simulink model "gm_Qiu_YQ"  (R2020a)
settings: Solver=FixedStepDiscrete  StartTime=0.0  StopTime=1.5  RelTol=1e-3
undefined symbols (not defined in the file or in its folder): N
libraries: dspsrcs4 x1
settings Model: SimulationMode=accelerator  Creator=huawei  LastModifiedBy=huawei
settings DataIOCC: SaveOutput=off  SaveTime=off
settings OptimizationCC: BlockReduction=off  ConditionallyExecuteInputs=off  DefaultParameterBehavior=Inlined
settings DebuggingCC: SignalRangeChecking=error  AlgebraicLoopMsg=error  InheritedTsInSrcMsg=none  SingleTaskRateTransMsg=error  ParameterDowncastMsg=none  ParameterOverflowMsg=none  ParameterPrecisionLossMsg=none  ArithmeticOperatorsInVariantConditions=warning
settings HardwareCC: ProdBitPerPointer=32  ProdBitPerSizeT=32  ProdBitPerPtrDiffT=32  ProdLargestAtomicFloat=None  ProdIntDivRoundTo=Undefined  ProdEndianess=Unspecified  ProdWordSize=32  ProdHWDeviceType=ASIC/FPGA->ASIC/FPGA  TargetBitPerPointer=64  TargetBitPerSizeT=64  TargetBitPerPtrDiffT=64  TargetLongLongMode=on  TargetIntDivRoundTo=Zero  TargetEndianess=LittleEndian  TargetWordSize=64  TargetHWDeviceType=Custom Processor->MATLAB Host Computer  ProdEqTarget=off
settings SFSimCC: CustomCodeUndefinedFunction=UseInterfaceOnly

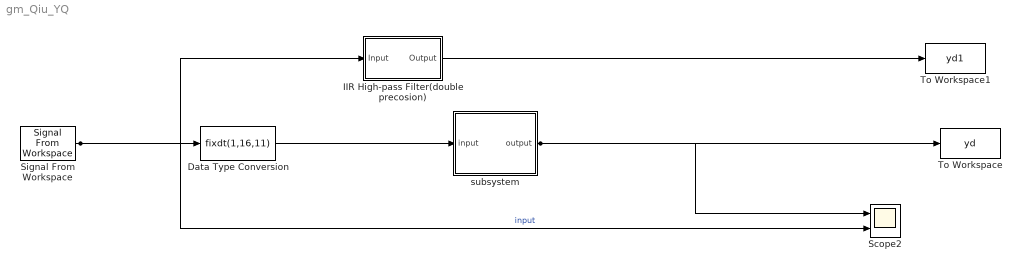
== system gm_Qiu_YQ ==
  Data Type Conversion : DataTypeConversion  OutDataTypeStr=fixdt(1,16,11)  RndMeth=Convergent
  IIR High-pass Filter(double precosion) : Subsystem  Tag=FilterWizardSubSystem
      settings: ErrorFcn=dspFilterRealizedInBasicElemsAlgLoopErrFcnCallback
  Scope2 : Scope  NumInputPorts=2
  Signal From Workspace : dspsrcs4/Signal From Workspace  X=x  Ts=1/N  nsamps=1  OutputAfterFinalValue=Setting to zero  ignoreOrWarnInputAndFrameLengths=off  OutputFrames=off
  To Workspace : ToWorkspace  VariableName=yd  SaveFormat=Timeseries  SampleTime=-1
  To Workspace1 : ToWorkspace  VariableName=yd1  SaveFormat=Timeseries  SampleTime=-1
  subsystem : Subsystem
  wires:
  Data Type Conversion/1 -> subsystem/1(input)
  subsystem/1(output) -> To Workspace/1, Scope2/1
  IIR High-pass Filter(double precosion)/1(Output) -> To Workspace1/1
  Signal From Workspace/1 -> Data Type Conversion/1, IIR High-pass Filter(double precosion)/1(Input), Scope2/2  "input"

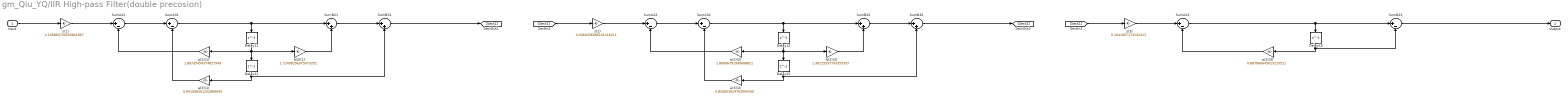
== system gm_Qiu_YQ/IIR High-pass Filter(double precosion) ==
  Input : Inport
  Delay{11..13,21..22} (5 alike) : Delay  DelayLength=1  InitialCondition=0
  SumA{21..23,31..32} (5 alike) : Sum  Inputs=|+-  RndMeth=Nearest  SaturateOnIntegerOverflow=on  OutDataTypeStr=Inherit: Same as first input
  SumB{21..22,31..32} (4 alike) : Sum  Inputs=|++  RndMeth=Nearest  SaturateOnIntegerOverflow=on  OutDataTypeStr=Inherit: Same as first input
  SumB23 : Sum  Inputs=|+-  RndMeth=Nearest  SaturateOnIntegerOverflow=on  OutDataTypeStr=Inherit: Same as first input
  a(2)(1) : Gain  Gain=1.88735454374827949  ParamDataTypeStr=double  RndMeth=Nearest  SaturateOnIntegerOverflow=on  OutDataTypeStr=Inherit: Same as input
  a(2)(2) : Gain  Gain=1.80696791990688821  ParamDataTypeStr=double  RndMeth=Nearest  SaturateOnIntegerOverflow=on  OutDataTypeStr=Inherit: Same as input
  a(2)(3) : Gain  Gain=0.887060645613220511  ParamDataTypeStr=double  RndMeth=Nearest  SaturateOnIntegerOverflow=on  OutDataTypeStr=Inherit: Same as input
  a(3)(1) : Gain  Gain=0.941058301252869045  ParamDataTypeStr=double  RndMeth=Nearest  SaturateOnIntegerOverflow=on  OutDataTypeStr=Inherit: Same as input
  a(3)(2) : Gain  Gain=0.835803624763594266  ParamDataTypeStr=double  RndMeth=Nearest  SaturateOnIntegerOverflow=on  OutDataTypeStr=Inherit: Same as input
  b(2)(1) : Gain  Gain=1.72499296375073352  ParamDataTypeStr=double  RndMeth=Nearest  SaturateOnIntegerOverflow=on  OutDataTypeStr=Inherit: Same as input
  b(2)(2) : Gain  Gain=1.38125597793355337  ParamDataTypeStr=double  RndMeth=Nearest  SaturateOnIntegerOverflow=on  OutDataTypeStr=Inherit: Same as input
  s(1) : Gain  Gain=0.105863730533801867  ParamDataTypeStr=double  RndMeth=Nearest  SaturateOnIntegerOverflow=on  OutDataTypeStr=Inherit: Same as input
  s(2) : Gain  Gain=0.0466036096161416211  ParamDataTypeStr=double  RndMeth=Nearest  SaturateOnIntegerOverflow=on  OutDataTypeStr=Inherit: Same as input
  s(3) : Gain  Gain=0.1041667174132411  ParamDataTypeStr=double  RndMeth=Nearest  SaturateOnIntegerOverflow=on  OutDataTypeStr=Inherit: Same as input
  Output : Outport
  wires:
  Delay13/1 -> SumB23/2, a(2)(3)/1
  a(2)(3)/1 -> SumA23/2
  SumB23/1 -> Output/1
  SumA23/1 -> Delay13/1, SumB23/1
  s(3)/1 -> SumA23/1
  [Sect2] -> s(3)/1
  Delay22/1 -> SumB32/2, a(3)(2)/1
  a(3)(2)/1 -> SumA32/2
  b(2)(2)/1 -> SumB22/2
  Delay12/1 -> Delay22/1, b(2)(2)/1, a(2)(2)/1
  a(2)(2)/1 -> SumA22/2
  SumB32/1 -> [Sect2]
  SumB22/1 -> SumB32/1
  SumA32/1 -> Delay12/1, SumB22/1
  SumA22/1 -> SumA32/1
  s(2)/1 -> SumA22/1
  [Sect1] -> s(2)/1
  Delay21/1 -> SumB31/2, a(3)(1)/1
  a(3)(1)/1 -> SumA31/2
  b(2)(1)/1 -> SumB21/2
  Delay11/1 -> Delay21/1, b(2)(1)/1, a(2)(1)/1
  a(2)(1)/1 -> SumA21/2
  SumB31/1 -> [Sect1]
  SumB21/1 -> SumB31/1
  SumA31/1 -> Delay11/1, SumB21/1
  SumA21/1 -> SumA31/1
  s(1)/1 -> SumA21/1
  Input/1 -> s(1)/1

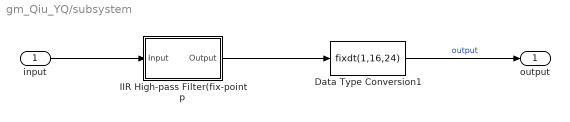
== system gm_Qiu_YQ/subsystem ==
  input : Inport
  Data Type Conversion1 : DataTypeConversion  OutDataTypeStr=fixdt(1,16,24)
  IIR High-pass Filter(fix-point p : Subsystem  Tag=FilterWizardSubSystem
      settings: ErrorFcn=dspFilterRealizedInBasicElemsAlgLoopErrFcnCallback
  output : Outport
  wires:
  Data Type Conversion1/1 -> output/1  "output"
  input/1 -> IIR High-pass Filter(fix-point p/1(Input)
  IIR High-pass Filter(fix-point p/1(Output) -> Data Type Conversion1/1

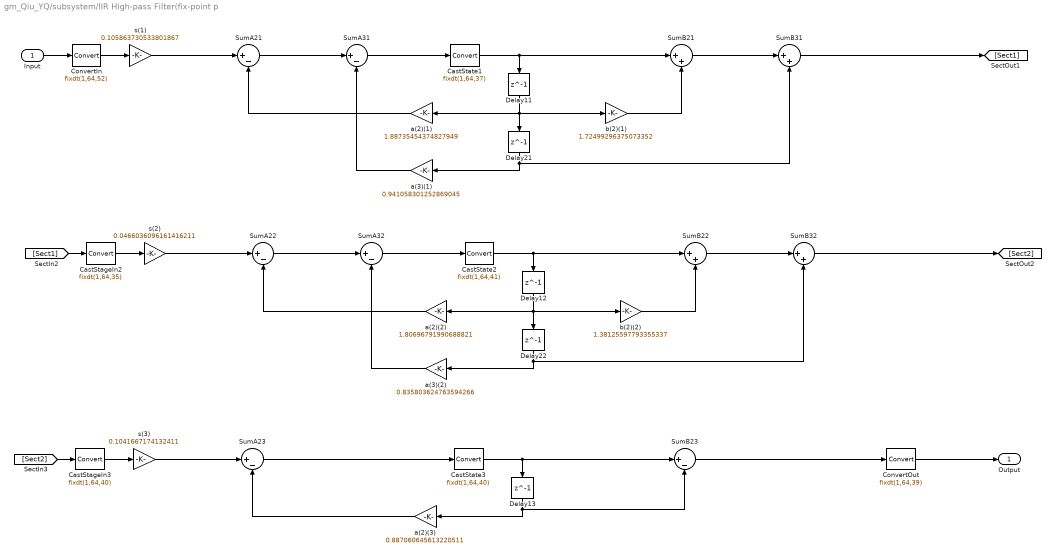
== system gm_Qiu_YQ/subsystem/IIR High-pass Filter(fix-point p ==
  Input : Inport  OutDataTypeStr=fixdt(1,16,11)  LockScale=on
  CastStageIn2 : DataTypeConversion  OutDataTypeStr=fixdt(1,64,35)  RndMeth=Convergent
  CastStageIn3 : DataTypeConversion  OutDataTypeStr=fixdt(1,64,40)  RndMeth=Convergent
  CastState1 : DataTypeConversion  OutDataTypeStr=fixdt(1,64,37)  RndMeth=Convergent
  CastState2 : DataTypeConversion  OutDataTypeStr=fixdt(1,64,41)  RndMeth=Convergent
  CastState3 : DataTypeConversion  OutDataTypeStr=fixdt(1,64,40)  RndMeth=Convergent
  ConvertIn : DataTypeConversion  OutDataTypeStr=fixdt(1,64,52)  RndMeth=Nearest  SaturateOnIntegerOverflow=on
  ConvertOut : DataTypeConversion  OutDataTypeStr=fixdt(1,64,39)  RndMeth=Convergent
  Delay{11..13,21..22} (5 alike) : Delay  DelayLength=1  InitialCondition=0
  SumA21 : Sum  Inputs=|+-  AccumDataTypeStr=fixdt(1,64,53)  OutDataTypeStr=fixdt(1,64,33)  RndMeth=Convergent
  SumA22 : Sum  Inputs=|+-  AccumDataTypeStr=fixdt(1,64,39)  OutDataTypeStr=fixdt(1,64,37)  RndMeth=Convergent
  SumA23 : Sum  Inputs=|+-  AccumDataTypeStr=fixdt(1,64,39)  OutDataTypeStr=fixdt(1,64,39)  RndMeth=Convergent
  SumA31 : Sum  Inputs=|+-  AccumDataTypeStr=fixdt(1,64,33)  OutDataTypeStr=fixdt(1,64,34)  RndMeth=Convergent
  SumA32 : Sum  Inputs=|+-  AccumDataTypeStr=fixdt(1,64,37)  OutDataTypeStr=fixdt(1,64,38)  RndMeth=Convergent
  SumB21 : Sum  Inputs=|++  AccumDataTypeStr=fixdt(1,64,33)  OutDataTypeStr=fixdt(1,64,33)  RndMeth=Convergent
  SumB22 : Sum  Inputs=|++  AccumDataTypeStr=fixdt(1,64,38)  OutDataTypeStr=fixdt(1,64,38)  RndMeth=Convergent
  SumB23 : Sum  Inputs=|+-  AccumDataTypeStr=fixdt(1,64,39)  OutDataTypeStr=fixdt(1,64,39)  RndMeth=Convergent
  SumB31 : Sum  Inputs=|++  AccumDataTypeStr=fixdt(1,64,35)  OutDataTypeStr=fixdt(1,64,34)  RndMeth=Convergent
  SumB32 : Sum  Inputs=|++  AccumDataTypeStr=fixdt(1,64,38)  OutDataTypeStr=fixdt(1,64,37)  RndMeth=Convergent
  a(2)(1) : Gain  Gain=1.88735454374827949  ParamDataTypeStr=fixdt(0,16,15)  OutDataTypeStr=fixdt(1,64,32)  RndMeth=Convergent
  a(2)(2) : Gain  Gain=1.80696791990688821  ParamDataTypeStr=fixdt(0,16,15)  OutDataTypeStr=fixdt(1,32,35)  RndMeth=Convergent
  a(2)(3) : Gain  Gain=0.887060645613220511  ParamDataTypeStr=fixdt(0,16,16)  OutDataTypeStr=fixdt(1,32,38)  RndMeth=Convergent
  a(3)(1) : Gain  Gain=0.941058301252869045  ParamDataTypeStr=fixdt(0,16,16)  OutDataTypeStr=fixdt(1,64,34)  RndMeth=Convergent
  a(3)(2) : Gain  Gain=0.835803624763594266  ParamDataTypeStr=fixdt(0,16,16)  OutDataTypeStr=fixdt(1,32,36)  RndMeth=Convergent
  b(2)(1) : Gain  Gain=1.72499296375073352  ParamDataTypeStr=fixdt(0,16,15)  OutDataTypeStr=fixdt(1,64,34)  RndMeth=Convergent
  b(2)(2) : Gain  Gain=1.38125597793355337  ParamDataTypeStr=fixdt(0,16,15)  OutDataTypeStr=fixdt(1,32,35)  RndMeth=Convergent
  s(1) : Gain  Gain=0.105863730533801867  ParamDataTypeStr=fixdt(0,16,19)  OutDataTypeStr=fixdt(1,64,54)  RndMeth=Convergent
  s(2) : Gain  Gain=0.0466036096161416211  ParamDataTypeStr=fixdt(0,16,20)  OutDataTypeStr=fixdt(1,64,41)  RndMeth=Convergent
  s(3) : Gain  Gain=0.1041667174132411  ParamDataTypeStr=fixdt(0,16,19)  OutDataTypeStr=fixdt(1,64,42)  RndMeth=Convergent
  Output : Outport
  wires:
  CastStageIn3/1 -> s(3)/1
  ConvertOut/1 -> Output/1
  Delay13/1 -> SumB23/2, a(2)(3)/1
  a(2)(3)/1 -> SumA23/2
  SumB23/1 -> ConvertOut/1
  CastState3/1 -> Delay13/1, SumB23/1
  SumA23/1 -> CastState3/1
  s(3)/1 -> SumA23/1
  [Sect2] -> CastStageIn3/1
  CastStageIn2/1 -> s(2)/1
  Delay22/1 -> SumB32/2, a(3)(2)/1
  a(3)(2)/1 -> SumA32/2
  b(2)(2)/1 -> SumB22/2
  Delay12/1 -> Delay22/1, b(2)(2)/1, a(2)(2)/1
  a(2)(2)/1 -> SumA22/2
  SumB32/1 -> [Sect2]
  SumB22/1 -> SumB32/1
  CastState2/1 -> Delay12/1, SumB22/1
  SumA32/1 -> CastState2/1
  SumA22/1 -> SumA32/1
  s(2)/1 -> SumA22/1
  [Sect1] -> CastStageIn2/1
  ConvertIn/1 -> s(1)/1
  Delay21/1 -> SumB31/2, a(3)(1)/1
  a(3)(1)/1 -> SumA31/2
  b(2)(1)/1 -> SumB21/2
  Delay11/1 -> Delay21/1, b(2)(1)/1, a(2)(1)/1
  a(2)(1)/1 -> SumA21/2
  SumB31/1 -> [Sect1]
  SumB21/1 -> SumB31/1
  CastState1/1 -> Delay11/1, SumB21/1
  SumA31/1 -> CastState1/1
  SumA21/1 -> SumA31/1
  s(1)/1 -> SumA21/1
  Input/1 -> ConvertIn/1
